simulink model "three_phase_full_converter"  (R2024a)
settings: Solver=VariableStepAuto  StartTime=0.0  StopTime=0.1  RelTol=1e-3
undefined symbols (not defined in the file): a
libraries: spsThyristorLib x6, spsACVoltageSourceLib x3, spsMeanLib x2, spsRMSLib x2, dspstat3 x2, spsGroundLib x1, spsCurrentMeasurementLib x1, spsVoltageMeasurementLib x1, spsSeriesRLCBranchLib x1, spsThreePhaseVIMeasurementLib x1, sps_lib x1
settings Model: Creator=Asus  LastModifiedBy=Asus

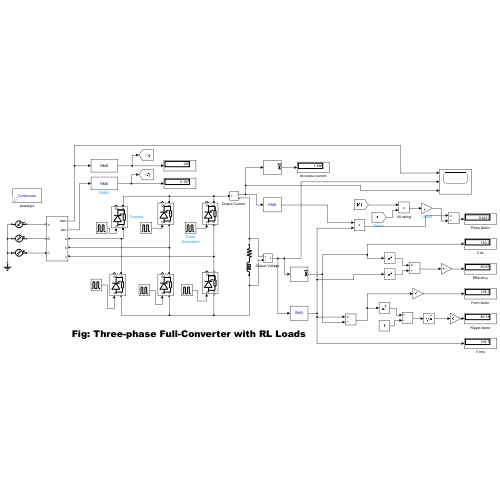
[thumbnail: Simulink's stored preview of the top-level diagram]
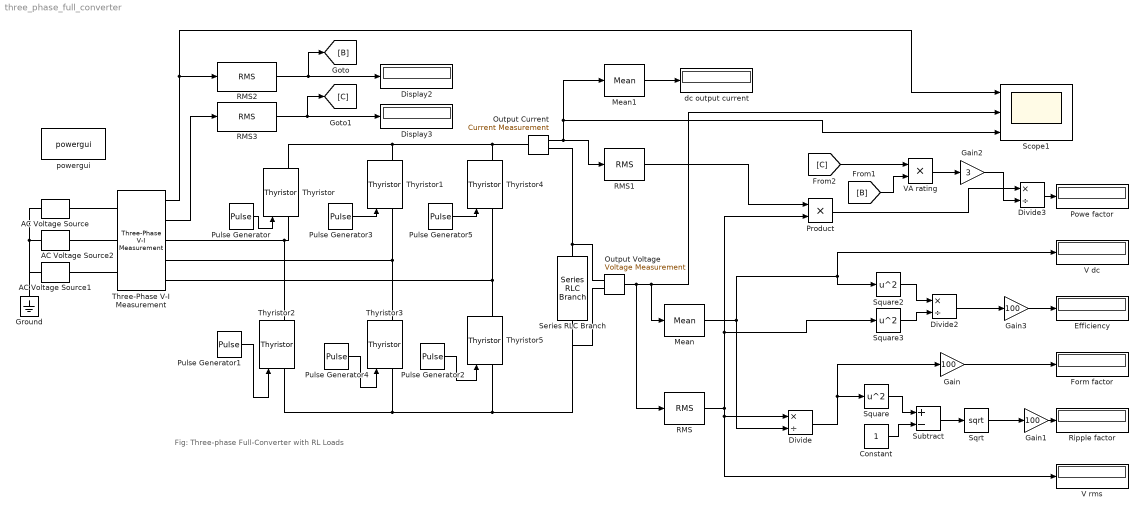
== system three_phase_full_converter ==
  note: Fig: Three-phase Full-Converter with RL Loads
  AC Voltage Source : spsACVoltageSourceLib/AC Voltage Source  Amplitude=120*sqrt(2)  Phase=0  Frequency=50  SampleTime=0  Measurements=Voltage  BusType=swing  Pref=10e3  Qref=0  Qmin=-inf  Qmax=+inf
  AC Voltage Source1 : spsACVoltageSourceLib/AC Voltage Source  Amplitude=120*sqrt(2)  Phase=-240  Frequency=50  SampleTime=0  Measurements=Voltage  BusType=swing  Pref=10e3  Qref=0  Qmin=-inf  Qmax=+inf
  AC Voltage Source2 : spsACVoltageSourceLib/AC Voltage Source  Amplitude=120*sqrt(2)  Phase=-120  Frequency=50  SampleTime=0  Measurements=Voltage  BusType=swing  Pref=10e3  Qref=0  Qmin=-inf  Qmax=+inf
  Constant : Constant
  Display2 : Display
  Display3 : Display
  Divide : Product  Inputs=*/
  Divide2 : Product  Inputs=*/
  Divide3 : Product  Inputs=*/
  "Efficiency " : Display
  Form factor : Display
  Gain : Gain  Gain=100
  Gain1 : Gain  Gain=100
  Gain2 : Gain  Gain=3
  Gain3 : Gain  Gain=100
  Ground : spsGroundLib/Ground  LConnTagsString=a
  Mean : spsMeanLib/Mean  Freq=60  Vinit=0  Ts=0
  Mean1 : spsMeanLib/Mean  Freq=60  Vinit=0  Ts=0
  "Output Current " : spsCurrentMeasurementLib/Current Measurement  PhasorSimulation=off  OutputType=Complex  PSBequivalent=0
  "Output Voltage " : spsVoltageMeasurementLib/Voltage Measurement  PhasorSimulation=off  OutputType=Complex  PSBequivalent=0
  Powe factor : Display
  Product : Product
  Pulse Generator : DiscretePulseGenerator  PulseType=Time based  Period=0.02  PulseWidth=5  PhaseDelay=a*0.02/360
  Pulse Generator1 : DiscretePulseGenerator  PulseType=Time based  Period=0.02  PulseWidth=5  PhaseDelay=(a+180)*0.02/360
  Pulse Generator2 : DiscretePulseGenerator  PulseType=Time based  Period=0.02  PulseWidth=5  PhaseDelay=(a+60)*0.02/360
  Pulse Generator3 : DiscretePulseGenerator  PulseType=Time based  Period=0.02  PulseWidth=5  PhaseDelay=(a+120)*0.02/360
  Pulse Generator4 : DiscretePulseGenerator  PulseType=Time based  Period=0.02  PulseWidth=5  PhaseDelay=(a+300)*0.02/360
  Pulse Generator5 : DiscretePulseGenerator  PulseType=Time based  Period=0.02  PulseWidth=5  PhaseDelay=(a+240)*0.02/360
  RMS : spsRMSLib/RMS  TrueRMS=on  Freq=60  RMSInit=120  Ts=0
  RMS1 : spsRMSLib/RMS  TrueRMS=on  Freq=60  RMSInit=120  Ts=0
  RMS2 : dspstat3/RMS  run=off  directionMode=Each column  dimension=1  InputProcessing=Columns as channels (frame based)  reset_popup=None
  RMS3 : dspstat3/RMS  run=off  directionMode=Each column  dimension=1  InputProcessing=Columns as channels (frame based)  reset_popup=None
  Ripple factor : Display
  Scope1 : Scope  NumInputPorts=3
  Series RLC Branch : spsSeriesRLCBranchLib/Series RLC Branch  LConnTagsString=__new0  RConnTagsString=__new0  BranchType=RL  Resistance=100  Inductance=0.1  SetiL0=off  InitialCurrent=0  Capacitance=1e-6  Setx0=off  InitialVoltage=0  Measurements=None
  Sqrt : Sqrt
  Square : Math  Operator=square  SignedPower=on
  Square2 : Math  Operator=square  SignedPower=on
  Square3 : Math  Operator=square  SignedPower=on
  Subtract : Sum  Inputs=+-
  Three-Phase V-I Measurement : spsThreePhaseVIMeasurementLib/Three-Phase V-I Measurement  VoltageMeasurement=phase-to-ground  SetLabelV=off  LabelV=Vabc  Vpu=off  VpuLL=off  CurrentMeasurement=yes  SetLabelI=off  LabelI=Iabc  Ipu=off  Pbase=100e6  Vbase=500e3  OutputType=Complex  PhasorSimulation=off  PSBequivalent=0
  Thyristor{,1..5} (6 alike) : spsThyristorLib/Thyristor  Ron=0.001  Lon=0  Vf=0.8  IC=0  Rs=500  Cs=250e-9  Measurements=on
  V dc : Display
  V rms : Display
  VA rating : Product
  dc output current : Display
  powergui : sps_lib/powergui  Priority=1  SimulationMode=Continuous  SampleTime=50e-6  frequency=60  Iterations=50  frequencyindice=50  Pbase=100e6  ErrMax=1e-4  UnitsV=kV  UnitsW=MW  buscounter=0  FunctionMessages=off  echomessages=off  EnableUseOfTLC=off  CurrentSourceSwitches=off  DisableSnubberDevices=off  DisableRonSwitches=off  DisableVfSwitches=off  DisplayEquations=off  AutomaticDiscreteSolvers=off  SolverType=Tustin/Backward Euler (TBE)  Interpol=off  ExternalGateDelay=off  methode=off  Ts=100  x0status=blocks  SPID=on  SwTol=0  HookPort=off  NonlinearTolerance=1e-4  nMaxIteration=100  ContinueOnMaxIteration=off  RestoreLinks=warning  ResistiveCurrentMeasurement=off  Frange=[0:2:500]  Ylog=off  Xlog=on  ShowGrid=off  save=off  variable=ZData  structure=0  ZoomFFT=off  StartTime=0.0  cycles=1  DisplayStyle=1  fundamental=60  FreqAxis=off  MaxFrequency=1000  frequencyindicesteady=1  RmsSteady=1  display=off
  wires:
  Square3/1 -> Divide2/2
  Pulse Generator5/1 -> Thyristor4/1
  Product/1 -> Divide3/1
  Divide2/1 -> Gain3/1
  Gain/1 -> Form factor/1
  Mean/1 -> Divide/2, V dc/1, Square2/1
  Three-Phase V-I Measurement/2 -> RMS3/1
  RMS/1 -> Divide/1, V rms/1, Product/2, Square3/1
  Square/1 -> Subtract/1
  [C] -> VA rating/1
  Three-Phase V-I Measurement/1 -> Scope1/1, RMS2/1
  Subtract/1 -> Sqrt/1
  Pulse Generator1/1 -> Thyristor2/1
  Pulse Generator/1 -> Thyristor/1
  Sqrt/1 -> Gain1/1
  Gain3/1 -> "Efficiency "/1
  Pulse Generator4/1 -> Thyristor3/1
  Gain2/1 -> Divide3/2
  RMS1/1 -> Product/1
  VA rating/1 -> Gain2/1
  Divide/1 -> Gain/1, Square/1
  RMS3/1 -> [C], Display3/1
  Square2/1 -> Divide2/1
  Constant/1 -> Subtract/2
  Mean1/1 -> dc output current/1
  "Output Current "/1 -> Mean1/1, Scope1/3, RMS1/1
  "Output Voltage "/1 -> Scope1/2, Mean/1, RMS/1
  Pulse Generator2/1 -> Thyristor5/1
  Pulse Generator3/1 -> Thyristor1/1
  Gain1/1 -> Ripple factor/1
  RMS2/1 -> [B], Display2/1
  Divide3/1 -> Powe factor/1
  [B] -> VA rating/2
  connections:
  Thyristor4/RConn1 -- "Output Current "/LConn1 -- Thyristor/RConn1 -- Thyristor1/RConn1
  Three-Phase V-I Measurement/RConn2 -- Thyristor3/RConn1 -- Thyristor1/LConn1
  Thyristor5/LConn1 -- "Output Voltage "/LConn2 -- Series RLC Branch/RConn1 -- Thyristor2/LConn1 -- Thyristor3/LConn1
  Three-Phase V-I Measurement/RConn3 -- Thyristor5/RConn1 -- Thyristor4/LConn1
  Series RLC Branch/LConn1 -- "Output Current "/RConn1 -- "Output Voltage "/LConn1
  AC Voltage Source2/LConn1 -- AC Voltage Source/LConn1 -- Ground/LConn1 -- AC Voltage Source1/LConn1
  Three-Phase V-I Measurement/RConn1 -- Thyristor2/RConn1 -- Thyristor/LConn1
  Three-Phase V-I Measurement/LConn2 -- AC Voltage Source2/RConn1
  AC Voltage Source1/RConn1 -- Three-Phase V-I Measurement/LConn3
  AC Voltage Source/RConn1 -- Three-Phase V-I Measurement/LConn1
